simulink model "xinhaochazheng"  (R2022b)
settings: Solver=VariableStepAuto  StartTime=0.0  StopTime=10.0  RelTol=1e-3
undefined symbols (not defined in the file or in its folder): CRB, ENV
settings Model: Creator=22428  LastModifiedBy=12045

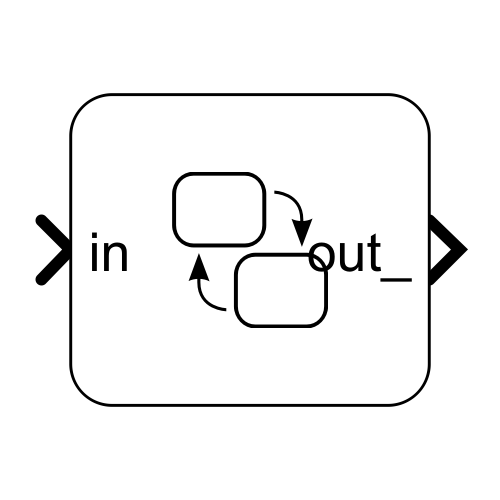
[thumbnail: Simulink's stored preview of the top-level diagram]
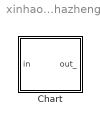
== system xinhaochazheng ==
  Chart : Stateflow chart  TreatAsAtomicUnit=on

== stateflow chart xinhaochazheng/Chart ==
  state function calc(in) [group]
    (default) -> (junction 7)
    (junction 7) -> (junction 8) : {d_in=in-ink1;}
    (junction 8) -> (junction 9) [order 1] : [d_in~=0]
    (junction 8) -> (junction 11) [order 2]
    (junction 9) -> (junction 10) : {
        | outk1=ink1;
        | d_out=d_in*CRB/ENV;
        | step=0;
        | }
    (junction 10) -> (junction 11)
    (junction 11) -> (junction 12)
    (junction 12) -> (junction 13) [order 1] : [step<(ENV/CRB-1)]
    (junction 12) -> (junction 37) [order 2] : {
        | out_=in;
        | }
    (junction 13) -> (junction 14) : {
        | step = step + 1;
        | out_=outk1+d_out;
        | }
    (junction 14) -> (junction 16) [order 1] : [d_out<0]
    (junction 14) -> (junction 18) [order 2]
    (junction 16) -> (junction 17) : {
        | out_=max(out_,in);
        | }
    (junction 17) -> (junction 18)
    (junction 18) -> (junction 32)
    (junction 32) -> (junction 33) [order 1] : [d_out>0]
    (junction 32) -> (junction 35) [order 2]
    (junction 33) -> (junction 34) : {
        | out_=min(out_,in);
        | }
    (junction 34) -> (junction 35)
    (junction 35) -> (junction 36)
    (junction 36) -> (junction 37)
    (junction 37) -> (junction 38) : {
        | ink1=in;
        | outk1=out_;
        | }
  data: ink1 local; outk1 local; step local; d_out local; d_in local; CRB parameter double size=10; ENV parameter double size=10; out_ output; in input
